simulink model "NDT_Localization"  (R2022a)
settings: Solver=FixedStepAuto  StartTime=0.0  StopTime=10.0  RelTol=1e-3
model workspace (MAT data in the model file):
  SL_ROS_VariableLengthArrays_MaxSizes.CommonInfo.ArrayTruncateAction = 'EmitWarning'
  SL_ROS_VariableLengthArrays_MaxSizes.MsgTypeMap = containers.Map
  SL_ROS_VariableLengthArrays_MaxSizes.MsgTypeMap.serialization.keys = {'sensor_msgs/PointCloud2'}
  SL_ROS_VariableLengthArrays_MaxSizes.MsgTypeMap.serialization.values{1}(1).PropertyName = 'data'
  SL_ROS_VariableLengthArrays_MaxSizes.MsgTypeMap.serialization.values{1}(1).DataType = 'uint8'
  SL_ROS_VariableLengthArrays_MaxSizes.MsgTypeMap.serialization.values{1}(1).MaxLength = 1760000
  SL_ROS_VariableLengthArrays_MaxSizes.MsgTypeMap.serialization.values{1}(2).PropertyName = 'fields'
  SL_ROS_VariableLengthArrays_MaxSizes.MsgTypeMap.serialization.values{1}(2).DataType = 'sensor_msgs/PointField'
  SL_ROS_VariableLengthArrays_MaxSizes.MsgTypeMap.serialization.values{1}(2).MaxLength = 16
  SL_ROS_VariableLengthArrays_MaxSizes.MsgTypeMap.serialization.uniformity = 0
  SL_ROS_VariableLengthArrays_MaxSizes.MsgTypeMap.serialization.keyType = 'char'
  SL_ROS_VariableLengthArrays_MaxSizes.MsgTypeMap.serialization.valueType = 'any'
undefined symbols (not defined in the file or in its folder): null
libraries: ros2lib x9, robotlib x8, simulink x1
(part 1 of 12)
settings Model: Creator=takumi onozawa  LastModifiedBy=takum
settings OptimizationCC: EnhancedBackFolding=on  PassReuseOutputArgsAs=Individual arguments  ZeroExternalMemoryAtStartup=off  ZeroInternalMemoryAtStartup=off  MaxStackSize=64  OptimizeBlockOrder=speed  DifferentSizesBufferReuse=on  OptimizationCustomize=off  EfficientTunableParamExpr=on
settings DebuggingCC: ParameterTunabilityLossMsg=error  UnconnectedInputMsg=warning  UnconnectedOutputMsg=warning  UnconnectedLineMsg=warning
settings SFSimCC: MATLABDynamicMemAlloc=off
settings RTWCC: SystemTargetFile=ert.tlc  HardwareBoard=Robot Operating System 2 (ROS 2)  TLCOptions="-aInlineSetEventsForThisBaseRateFcn=TLC_FALSE -aSuppressMultiTaskScheduler=TLC_FALSE  -aRateBasedStepFcn=0"  TemplateMakefile=ert_default_tmf  Toolchain=Colcon Tools  TargetLang=C++  DLArmComputeVersion=19.05
settings CodeAppCC: ForceParamTrailComments=on  IgnoreCustomStorageClasses=off  OperatorAnnotations=on  SimulinkDataObjDesc=on  SFDataObjDesc=on  InsertBlockDesc=on
settings ERTTargetCC: CodeInterfacePackaging=C++ class  RootIOFormat=Structure reference

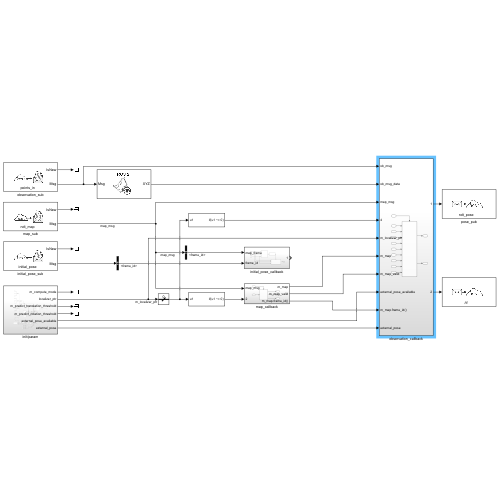
[thumbnail: Simulink's stored preview of the top-level diagram]
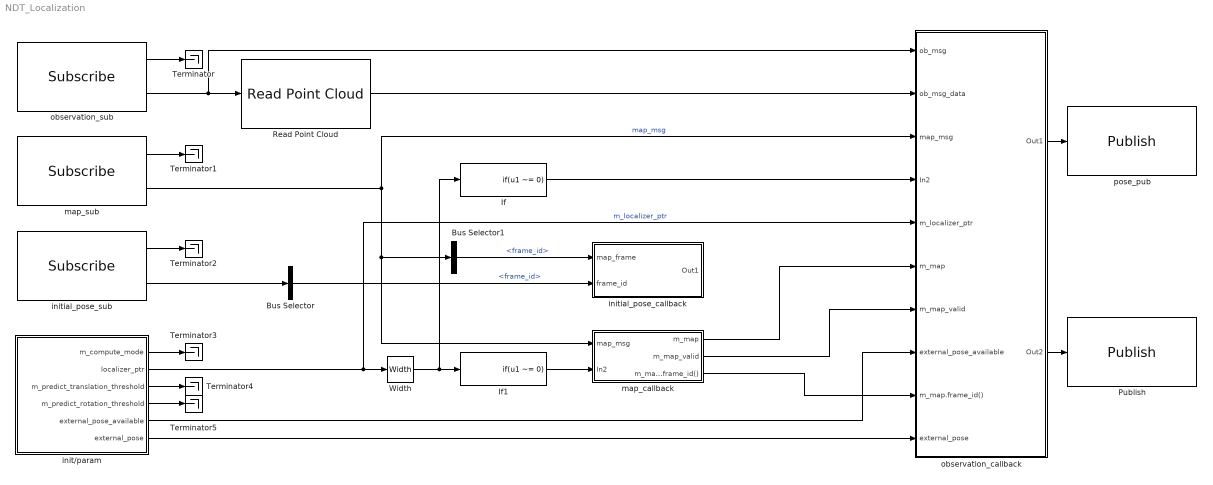
== system NDT_Localization ==
  Bus Selector : BusSelector  OutputSignals=header.frame_id
  Bus Selector1 : BusSelector  OutputSignals=header.frame_id
  If : If  IfExpression=u1 ~= 0  ShowElse=off
  If1 : If  IfExpression=u1 ~= 0  ShowElse=off
  Publish : ros2lib/Publish  topicSource=Specify your own  topic=/tf  messageType=geometry_msgs/Transform  QOSHistory=Keep last  QOSDepth=1  QOSReliability=Reliable  QOSDurability=Volatile
      settings: SourceProductBaseCode=RR
  Read Point Cloud : ros2lib/Read Point Cloud  MaximumPointCloudSize=[480, 640]  PreserveStructure=off  ShowRGBOutput=off  ShowIntensityOutput=off  ShowErrorCodeOutput=off  VariableSizeOutputs=off
      settings: SourceProductBaseCode=RR
  Terminator{,1..5} (6 alike) : Terminator
  Width : Width
  init/param : Subsystem
  initial_pose_callback : Subsystem
  initial_pose_sub : ros2lib/Subscribe  topicSource=Specify your own  topic=initial_pose  messageType=geometry_msgs/PoseWithCovarianceStamped  sampleTime=-1  QOSHistory=Keep last  QOSDepth=1  QOSReliability=Reliable  QOSDurability=Volatile
      settings: SourceProductBaseCode=RR
  map_callback : Subsystem
  map_sub : ros2lib/Subscribe  topicSource=Specify your own  topic=ndt_map  messageType=sensor_msgs/PointCloud2  sampleTime=-1  QOSHistory=Keep last  QOSDepth=1  QOSReliability=Reliable  QOSDurability=Volatile
      settings: SourceProductBaseCode=RR
  observation_callback : Subsystem
  observation_sub : ros2lib/Subscribe  topicSource=Specify your own  topic=points_in  messageType=sensor_msgs/PointCloud2  sampleTime=-1  QOSHistory=Keep last  QOSDepth=1  QOSReliability=Reliable  QOSDurability=Volatile
      settings: SourceProductBaseCode=RR
  pose_pub : ros2lib/Publish  topicSource=Specify your own  topic=ndt_pose  messageType=geometry_msgs/PoseWithCovarianceStamped  QOSHistory=Keep last  QOSDepth=1  QOSReliability=Reliable  QOSDurability=Volatile
      settings: SourceProductBaseCode=RR
  wires:
  observation_sub/1 -> Terminator/1
  map_sub/1 -> Terminator1/1
  initial_pose_sub/1 -> Terminator2/1
  observation_sub/2 -> observation_callback/1(ob_msg), Read Point Cloud/1
  init/param/2(localizer_ptr) -> observation_callback/5(m_localizer_ptr), Width/1  "m_localizer_ptr"
  initial_pose_sub/2 -> Bus Selector/1
  map_sub/2 -> observation_callback/3(map_msg), Bus Selector1/1, map_callback/1(map_msg)  "map_msg"
  Bus Selector1/1 -> initial_pose_callback/1(map_frame)  "<frame_id>"
  Bus Selector/1 -> initial_pose_callback/2(frame_id)  "<frame_id>"
  Read Point Cloud/1 -> observation_callback/2(ob_msg_data)
  If1/1 -> map_callback/2(In2)
  Width/1 -> If/1, If1/1
  If/1 -> observation_callback/4(In2)
  map_callback/2(m_map_valid) -> observation_callback/7(m_map_valid)
  init/param/5(external_pose_available) -> observation_callback/8(external_pose_available)
  init/param/6(external_pose) -> observation_callback/10(external_pose)
  observation_callback/1(Out1) -> pose_pub/1
  map_callback/1(m_map) -> observation_callback/6(m_map)
  observation_callback/2(Out2) -> Publish/1
  map_callback/3(m_map.frame_id()) -> observation_callback/9(m_map.frame_id())
  init/param/1(m_compute_mode) -> Terminator3/1
  init/param/3(m_predict_translation_threshold) -> Terminator4/1
  init/param/4(m_predict_rotation_threshold) -> Terminator5/1

== system NDT_Localization/init//param ==
  Blank Message : ros2lib/Blank Message  messageClass=Message  entityType=geometry_msgs/TransformStamped  messageType=geometry_msgs/TransformStamped  SampleTime=inf
      settings: SourceProductBaseCode=RR
  Bus Creator{,1..2,4..5,8..9} (7 alike) : BusCreator  Inputs=3
  Bus Creator10 : BusCreator  Inputs=4
  Bus Creator11 : BusCreator  Inputs=2
  Bus Creator12 : BusCreator  Inputs=4
  Bus Creator3 : BusCreator  Inputs=4
  Bus Creator6 : BusCreator  Inputs=6
  Bus Creator7 : BusCreator  Inputs=2
  Bus Selector : BusSelector  OutputSignals=header.stamp,header.frame_id_SL_Info,child_frame_id_SL_Info
  Constant{,1..5} (6 alike) : Constant  Value=0
  Constant6 : Constant
  Data Type Conversion : DataTypeConversion  OutDataTypeStr=double  SaturateOnIntegerOverflow=off  RndMeth=Floor
  If : If  NumInputs=5  IfExpression=u2 >= 0 & u1 >= u2 & (u3 >= 0.0 & u3 <= 1.0) & (u4 >= 0.0 & u4 <= 1.0) & u5 >= 1  ShowElse=off
  If Action Subsystem : Subsystem  TreatAsAtomicUnit=on
  MoreThuenteLineSearch : Subsystem
  String Constant : StringConstant  String="\"map\""
  String Constant1 : StringConstant  String="\"base_link\""
  String to ASCII : StringToASCII
  String to ASCII1 : StringToASCII
  guess_time_tolerance_ms : Constant  Value=5  OutDataTypeStr=uint64
  m_external_pose_available : Constant  Value=true  OutDataTypeStr=boolean
  map_capacity : Constant  Value=55000  OutDataTypeStr=uint32
  map_max_point_x : Constant  Value=130.0  OutDataTypeStr=int64
  map_max_point_y : Constant  Value=130.0  OutDataTypeStr=int64
  map_max_point_z : Constant  Value=3.0  OutDataTypeStr=int64
  map_min_point_x : Constant  Value=-130.0  OutDataTypeStr=int64
  map_min_point_y : Constant  Value=-130.0  OutDataTypeStr=int64
  map_min_point_z : Constant  Value=-3.0  OutDataTypeStr=int64
  map_voxel_size_x : Constant  Value=2.0  OutDataTypeStr=int64
  map_voxel_size_y : Constant  Value=2.0  OutDataTypeStr=int64
  map_voxel_size_z : Constant  Value=2.0  OutDataTypeStr=int64
  optimizer_options : Subsystem
  outlier_ratio : Constant  Value=0.55  OutDataTypeStr=double
  predict_rotation_threshold : Constant  Value=0.1
  predict_translation_threshold : Constant  Value=0.5
  scan_capacity : Constant  Value=55000  OutDataTypeStr=uint32
  step_max : Constant  Value=0.12
  step_min : Constant  Value=0.0001
  m_compute_mode : Outport
  localizer_ptr : Outport  Port=2
  m_predict_translation_threshold : Outport  Port=3
  m_predict_rotation_threshold : Outport  Port=4
  external_pose_available : Outport  Port=5
  external_pose : Outport  Port=6
  wires:
  map_voxel_size_x/1 -> Bus Creator2/1  "x"
  Bus Creator/1 -> Bus Creator3/1  "min_point"
  Data Type Conversion/1 -> If/5
  map_min_point_y/1 -> Bus Creator/2  "y"
  Bus Creator1/1 -> Bus Creator3/2  "max_point"
  MoreThuenteLineSearch/1(optimization_direction1) -> Bus Creator6/3
  Bus Creator4/1 -> Bus Creator8/1  "localizer_config"
  map_voxel_size_y/1 -> Bus Creator2/2  "y"
  Bus Creator2/1 -> Bus Creator3/3  "voxel_size"
  map_max_point_x/1 -> Bus Creator1/1  "x"
  step_max/1 -> If/1, Bus Creator6/1  "max_step"
  map_max_point_z/1 -> Bus Creator1/3  "z"
  MoreThuenteLineSearch/2(mu1) -> If/3, Bus Creator6/4
  step_min/1 -> If/2, Bus Creator6/2  "min_step"
  map_min_point_z/1 -> Bus Creator/3  "z"
  map_capacity/1 -> Bus Creator3/4  "capacity"
  MoreThuenteLineSearch/3(eta2) -> Bus Creator6/5, If/4
  optimizer_options/1(optimizer_options) -> Bus Creator7/2  "optimizer_options"
  outlier_ratio/1 -> Bus Creator8/3  "outlier_ratio"
  Bus Creator3/1 -> Bus Creator4/1  "map_config"
  predict_rotation_threshold/1 -> m_predict_rotation_threshold/1  "predict_rotation_threshold"
  map_max_point_y/1 -> Bus Creator1/2  "y"
  guess_time_tolerance_ms/1 -> Bus Creator4/3  "milliseconds"
  map_voxel_size_z/1 -> Bus Creator2/3  "z"
  predict_translation_threshold/1 -> m_predict_translation_threshold/1  "predict_translation_threshold"
  MoreThuenteLineSearch/4(max_iterations1) -> Bus Creator6/6, Data Type Conversion/1
  If/1 -> If Action Subsystem/Action
  Bus Creator6/1 -> Bus Creator7/1  "MoreThuenteLineSearch"
  Bus Creator7/1 -> Bus Creator8/2  "OptimizerT"
  scan_capacity/1 -> Bus Creator4/2  "capacity"
  map_min_point_x/1 -> Bus Creator/1  "x"
  Bus Creator8/1 -> localizer_ptr/1  "localizer_ptr"
  If Action Subsystem/1(m_compute_mode) -> m_compute_mode/1  "m_compute_mode"
  m_external_pose_available/1 -> external_pose_available/1
  Blank Message/1 -> Bus Selector/1
  Bus Selector/1 -> Bus Creator5/1  "<stamp>"
  String to ASCII/1 -> Bus Creator5/2  "frame_id"
  Bus Selector/2 -> Bus Creator5/3  "<frame_id_SL_Info>"
  Bus Creator5/1 -> Bus Creator12/1  "header"
  String to ASCII1/1 -> Bus Creator12/2  "child_frame_id"
  Bus Selector/3 -> Bus Creator12/3  "<child_frame_id_SL_Info>"
  Constant/1 -> Bus Creator9/1  "x"
  Constant1/1 -> Bus Creator9/2  "y"
  Constant2/1 -> Bus Creator9/3  "z"
  Bus Creator9/1 -> Bus Creator11/1  "translation"
  Constant3/1 -> Bus Creator10/1  "x"
  Constant4/1 -> Bus Creator10/2  "y"
  Constant5/1 -> Bus Creator10/3  "z"
  Constant6/1 -> Bus Creator10/4  "w"
  Bus Creator10/1 -> Bus Creator11/2  "rotation"
  Bus Creator11/1 -> Bus Creator12/4  "transform"
  String Constant1/1 -> String to ASCII1/1
  String Constant/1 -> String to ASCII/1
  Bus Creator12/1 -> external_pose/1  "external_pose"

== system NDT_Localization/initial_pose_callback ==
  map_frame : Inport
  frame_id : Inport  Port=2
  If1 : If  IfExpression=u1 ~= 0  ShowElse=off
  TimePointZero : Constant  Value=0
  canTransform : Subsystem
  lookupTransform : Subsystem  TreatAsAtomicUnit=on
  Out1 : Outport
  wires:
  lookupTransform/1(Out1) -> Out1/1
  canTransform/1(<frame_id>) -> If1/1
  If1/1 -> lookupTransform/Action
  map_frame/1 -> lookupTransform/1(target_frame), canTransform/1(target_frame)
  TimePointZero/1 -> lookupTransform/3(time), canTransform/3(time)
  frame_id/1 -> lookupTransform/2(source_frame), canTransform/2(source_frame)

== system NDT_Localization/map_callback ==
  map_msg : Inport
  In2 : Inport  Port=2
  check_localizer : Subsystem  TreatAsAtomicUnit=on
  m_map : Outport
  m_map_valid : Outport  Port=2
  m_map.frame_id() : Outport  Port=3
  wires:
  map_msg/1 -> check_localizer/1(map_msg)
  In2/1 -> check_localizer/Action
  check_localizer/1(m_map) -> m_map/1
  check_localizer/2(m_map_valid) -> m_map_valid/1
  check_localizer/3(m_map.frame_id()) -> m_map.frame_id()/1

== system NDT_Localization/observation_callback ==
  ob_msg : Inport
  ob_msg_data : Inport  Port=2
  map_msg : Inport  Port=3
  In2 : Inport  Port=4
  m_localizer_ptr : Inport  Port=5
  m_map : Inport  Port=6
  m_map_valid : Inport  Port=7
  external_pose_available : Inport  Port=8
  m_map.frame_id() : Inport  Port=9
  external_pose : Inport  Port=10
  check_localizer : Subsystem  TreatAsAtomicUnit=on
  Out1 : Outport
  Out2 : Outport  Port=2
  wires:
  In2/1 -> check_localizer/Action
  check_localizer/1(Out1) -> Out1/1
  m_map_valid/1 -> check_localizer/1(m_map_valid)
  ob_msg/1 -> check_localizer/2(ob_msg)
  map_msg/1 -> check_localizer/4(map_msg)
  external_pose_available/1 -> check_localizer/5(external_pose_available)
  external_pose/1 -> check_localizer/6(external_pose)
  m_map/1 -> check_localizer/7(m_map)
  check_localizer/2(Out2) -> Out2/1
  m_localizer_ptr/1 -> check_localizer/9(m_localizer_ptr)
  m_map.frame_id()/1 -> check_localizer/8(m_map.frame_id())
  ob_msg_data/1 -> check_localizer/3(ob_msg_data)

== system NDT_Localization/init//param/If Action Subsystem ==
  Action Port : ActionPort  ActionPortLabel=if(u2 >= 0 & u1 >= u2 & (u3 >= 0.0 & u3 <= 1.0) & (u4 >= 0.0 & u4 <= 1.0) & u5 >= 1)
  Bus Creator : BusCreator  Inputs=2
  set_jacobian : MATLAB Function  TreatAsAtomicUnit=on
  set_score : Constant  Value=0.0  OutDataTypeStr=single
  m_compute_mode : Outport
  wires:
  Bus Creator/1 -> m_compute_mode/1
  set_score/1 -> Bus Creator/1
  set_jacobian/1(jacobian) -> Bus Creator/2

== system NDT_Localization/init//param/MoreThuenteLineSearch ==
  eta : Constant  Value=0.1  OutDataTypeStr=double
  max_iterations : Constant  Value=10  OutDataTypeStr=int32
  mu : Constant  Value=0.0001
  optimization_direction : Constant  Value=1.0  OutDataTypeStr=double
  optimization_direction1 : Outport
  mu1 : Outport  Port=2
  eta2 : Outport  Port=3
  max_iterations1 : Outport  Port=4
  wires:
  optimization_direction/1 -> optimization_direction1/1  "optimization_direction"
  max_iterations/1 -> max_iterations1/1  "max_iterations"
  mu/1 -> mu1/1  "mu"
  eta/1 -> eta2/1  "eta"

== system NDT_Localization/init//param/optimizer_options ==
  Bus Creator5 : BusCreator  Inputs=4
  gradient_tolerance : Constant  Value=0.001  OutDataTypeStr=double
  max_iterations : Constant  Value=50  OutDataTypeStr=uint64
  parameter_tolerance : Constant  Value=0.001  OutDataTypeStr=double
  score_tolerance : Constant  Value=0.001  OutDataTypeStr=double
  optimizer_options : Outport
  wires:
  gradient_tolerance/1 -> Bus Creator5/4  "gradient_tolerance"
  parameter_tolerance/1 -> Bus Creator5/3  "parameter_tolerance"
  score_tolerance/1 -> Bus Creator5/2  "score_tolerance"
  Bus Creator5/1 -> optimizer_options/1  "optimizer_options"
  max_iterations/1 -> Bus Creator5/1  "max_iterations"

== system NDT_Localization/initial_pose_callback/canTransform ==
  target_frame : Inport
  source_frame : Inport  Port=2
  time : Inport  Port=3
  Bus Selector : BusSelector  OutputSignals=header.frame_id
  Constant : Constant  Value=true  OutDataTypeStr=boolean
  Constant1 : Constant  Value=false  OutDataTypeStr=boolean
  Constant2 : Constant  Value=false  OutDataTypeStr=boolean
  Constant3 : Constant  Value=false  OutDataTypeStr=boolean
  If1 : If  NumInputs=4  IfExpression=u1 == 1  ElseIfExpressions=u2 ~= 0, u3 == 0, u4 == 0
  Merge : Merge  Inputs=5
  String Compare : StringCompare
  else : Subsystem  TreatAsAtomicUnit=on
  lookupFrameNumber : Subsystem
  lookupFrameNumber1 : Subsystem
  true : Subsystem  TreatAsAtomicUnit=on
  true1 : Subsystem  TreatAsAtomicUnit=on
  true2 : Subsystem  TreatAsAtomicUnit=on
  true3 : Subsystem  TreatAsAtomicUnit=on
  warnFrameId : Subsystem
  <frame_id> : Outport
  wires:
  true/1(Out1) -> Merge/1
  true2/1(Out1) -> Merge/3
  Merge/1 -> <frame_id>/1
  else/1(Out1) -> Merge/5
  If1/5 -> else/Action
  Constant2/1 -> true2/1(In1)
  If1/3 -> true2/Action
  If1/4 -> true3/Action
  true1/1(Out1) -> Merge/2
  If1/2 -> true1/Action
  lookupFrameNumber1/1(source_id) -> else/2(source_id), If1/4  "source_id"
  Constant3/1 -> true3/1(In1)
  warnFrameId/1(Out1) -> If1/2
  String Compare/1 -> If1/1
  lookupFrameNumber/1(target_id) -> else/1(target_id), If1/3  "target_id"
  Constant1/1 -> true1/1(In1)
  Constant/1 -> true/1(In1)
  true3/1(Out1) -> Merge/4
  If1/1 -> true/Action
  target_frame/1 -> Bus Selector/1
  source_frame/1 -> lookupFrameNumber1/1(source_frame), warnFrameId/2(frame_id), String Compare/2
  time/1 -> else/3(time)
  Bus Selector/1 -> String Compare/1, warnFrameId/1(map_frame), lookupFrameNumber/1(target_frame)  "<frame_id>"

== system NDT_Localization/initial_pose_callback/lookupTransform ==
  target_frame : Inport
  source_frame : Inport  Port=2
  time : Inport  Port=3
  Action Port : ActionPort  ActionPortLabel=if(u1 ~= 0)
  If : If  IfExpression=u1 ~= 0
  String Compare : StringCompare
  Switch : Switch  Criteria=u2 > Threshold  SaturateOnIntegerOverflow=off  InputSameDT=off
  if_false : Subsystem  TreatAsAtomicUnit=on
  if_true : Subsystem  TreatAsAtomicUnit=on
  Out1 : Outport
  wires:
  source_frame/1 -> String Compare/2, if_false/2(source_frame), if_true/2(source_frame)
  String Compare/1 -> Switch/2, If/1
  If/1 -> if_true/Action
  If/2 -> if_false/Action
  time/1 -> if_false/3(time), if_true/3(time)
  target_frame/1 -> String Compare/1, if_false/1(target_frame), if_true/1(target_frame)
  if_true/1(identity) -> Switch/1
  if_false/1(output_transform) -> Switch/3
  Switch/1 -> Out1/1

== system NDT_Localization/map_callback/check_localizer ==
  map_msg : Inport
  Action Port : ActionPort  ActionPortLabel=if(u1 ~= 0)
  set_map : Subsystem
  m_map : Outport
  m_map_valid : Outport  Port=2
  m_map.frame_id() : Outport  Port=3
  wires:
  map_msg/1 -> set_map/1(msg)
  set_map/1(impl()) -> m_map/1
  set_map/2(m_map_valid) -> m_map_valid/1
  set_map/3(m_map.frame_id()) -> m_map.frame_id()/1

== system NDT_Localization/observation_callback/check_localizer ==
  m_map_valid : Inport
  ob_msg : Inport  Port=2
  ob_msg_data : Inport  Port=3
  map_msg : Inport  Port=4
  external_pose_available : Inport  Port=5
  external_pose : Inport  Port=6
  m_map : Inport  Port=7
  m_map.frame_id() : Inport  Port=8
  m_localizer_ptr : Inport  Port=9
  Action Port : ActionPort  ActionPortLabel=if(u1 ~= 0)
  Data Type Conversion : DataTypeConversion  OutDataTypeStr=uint8  SaturateOnIntegerOverflow=off  RndMeth=Floor
  If : If  IfExpression=u1 ~= 0  ShowElse=off
  If Action Subsystem : Subsystem  TreatAsAtomicUnit=on
  If Action Subsystem1 : Subsystem  TreatAsAtomicUnit=on
  If Action Subsystem2 : Subsystem  TreatAsAtomicUnit=on
  If1 : If  IfExpression=u1 ~= 0
  Merge : Merge
  Out1 : Outport
  Out2 : Outport  Port=2
  wires:
  m_map_valid/1 -> Data Type Conversion/1
  Data Type Conversion/1 -> If/1
  If/1 -> If Action Subsystem/Action
  ob_msg/1 -> If Action Subsystem/1(ob_msg)
  map_msg/1 -> If Action Subsystem/3(map_msg)
  external_pose_available/1 -> If Action Subsystem/4(external_pose_available)
  external_pose/1 -> If Action Subsystem/5(external_pose)
  m_map/1 -> If Action Subsystem/6(m_map)
  If Action Subsystem/3(Out2) -> If1/1
  If Action Subsystem1/1(Out1) -> Out1/1
  If1/1 -> If Action Subsystem1/Action
  If1/2 -> If Action Subsystem2/Action
  If Action Subsystem/2(pose_out) -> If Action Subsystem1/2(pose_out), Merge/1
  If Action Subsystem2/1(Out1) -> Merge/2
  If Action Subsystem/4(msg.header.stamp) -> If Action Subsystem2/1(msg.header.stamp)
  m_localizer_ptr/1 -> If Action Subsystem2/2(m_localizer_ptr), If Action Subsystem/8(localizer_ptr)
  Merge/1 -> Out2/1
  If Action Subsystem/1(msg) -> If Action Subsystem1/1(msg)
  m_map.frame_id()/1 -> If Action Subsystem/7(m_map.frame_id())
  ob_msg_data/1 -> If Action Subsystem/2(ob_msg_data)

== system NDT_Localization/initial_pose_callback/canTransform/else ==
  target_id : Inport
  source_id : Inport  Port=2
  time : Inport  Port=3
  Action Port : ActionPort  ActionPortLabel=else
  canTransformNoLock : Subsystem
  Out1 : Outport
  wires:
  source_id/1 -> canTransformNoLock/2(source_id)
  target_id/1 -> canTransformNoLock/1(target_id)
  canTransformNoLock/1(Out1) -> Out1/1
  time/1 -> canTransformNoLock/3(time)

== system NDT_Localization/initial_pose_callback/canTransform/lookupFrameNumber ==
  target_frame : Inport
  Cast : DataTypeConversion  SaturateOnIntegerOverflow=off  RndMeth=Floor
  target_id : Outport
  wires:
  target_frame/1 -> Cast/1
  Cast/1 -> target_id/1

== system NDT_Localization/initial_pose_callback/canTransform/lookupFrameNumber1 ==
  source_frame : Inport
  Cast : DataTypeConversion  SaturateOnIntegerOverflow=off  RndMeth=Floor
  source_id : Outport
  wires:
  Cast/1 -> source_id/1
  source_frame/1 -> Cast/1

== system NDT_Localization/initial_pose_callback/canTransform/true ==
  In1 : Inport
  Action Port : ActionPort  ActionPortLabel=if(u1 == 1)
  Out1 : Outport
  wires:
  In1/1 -> Out1/1

== system NDT_Localization/initial_pose_callback/canTransform/true1 ==
  In1 : Inport
  Action Port : ActionPort  ActionPortLabel=elseif(u2 ~= 0)
  Out1 : Outport
  wires:
  In1/1 -> Out1/1

== system NDT_Localization/initial_pose_callback/canTransform/true2 ==
  In1 : Inport
  Action Port : ActionPort  ActionPortLabel=elseif( u3 == 0)
  Out1 : Outport
  wires:
  In1/1 -> Out1/1

== system NDT_Localization/initial_pose_callback/canTransform/true3 ==
  In1 : Inport
  Action Port : ActionPort  ActionPortLabel=elseif( u4 == 0)
  Out1 : Outport
  wires:
  In1/1 -> Out1/1

== system NDT_Localization/initial_pose_callback/canTransform/warnFrameId ==
  map_frame : Inport
  frame_id : Inport  Port=2
  Add : Sum
  Add1 : Sum  Inputs=+++
  Cast : DataTypeConversion  OutDataTypeStr=boolean  SaturateOnIntegerOverflow=off  RndMeth=Floor
  Constant : Constant  OutDataTypeStr=double
  Display : Display
  If1 : If  IfExpression=u1 == 0  ShowElse=off
  If2 : If  IfExpression=u1 == 0  ShowElse=off
  If3 : If  ShowElse=off
  String Compare : StringCompare  CompareOption=First N characters
  String Compare1 : StringCompare  CompareOption=First N characters
  String Constant : StringConstant  String="\"\\\""
  String Length : StringLength
  String Length1 : StringLength
  false1 : Subsystem  TreatAsAtomicUnit=on
  false2 : Subsystem  TreatAsAtomicUnit=on
  false3 : Subsystem  TreatAsAtomicUnit=on
  Out1 : Outport
  wires:
  false2/1(Out1) -> Add1/2
  Constant/1 -> false1/1(In1), false3/1(In1), false2/1(In1)
  If1/1 -> false1/Action
  false3/1(Out1) -> Add1/3
  Add1/1 -> Cast/1
  String Constant/1 -> String Compare/2, String Compare1/1
  String Compare/1 -> Add/1
  String Compare1/1 -> Add/2
  Add/1 -> If3/1
  map_frame/1 -> String Compare/1, String Length/1
  false1/1(Out1) -> Add1/1
  frame_id/1 -> String Compare1/2, String Length1/1
  String Length/1 -> If1/1
  If3/1 -> false2/Action
  If2/1 -> false3/Action
  String Length1/1 -> If2/1
  Cast/1 -> Out1/1, Display/1

== system NDT_Localization/initial_pose_callback/lookupTransform/if_false ==
  target_frame : Inport
  source_frame : Inport  Port=2
  time : Inport  Port=3
  Action Port : ActionPort  ActionPortLabel=else
  Bus Creator : BusCreator  Inputs=3
  Bus Creator1 : BusCreator  Inputs=3
  Bus Creator2 : BusCreator  Inputs=2
  Bus Creator3 : BusCreator  Inputs=3
  Bus Creator4 : BusCreator  Inputs=4
  Bus Selector : BusSelector  OutputSignals=time,result_vec.x,result_vec.y,result_vec.z,result_quat.x,result_quat.y,result_quat.z,result_quat.w
  Constant : Constant
  Subsystem : Subsystem
  lookupFrameNumber : Subsystem
  lookupFrameNumber1 : Subsystem
  walkToTopParent : Subsystem  Commented=on
  output_transform : Outport
  wires:
  target_frame/1 -> lookupFrameNumber/1(target_frame), Bus Creator1/3  "frame_id"
  lookupFrameNumber/1(target_id) -> walkToTopParent/3(target_id)
  lookupFrameNumber1/1(source_id) -> walkToTopParent/4(source_id)
  time/1 -> walkToTopParent/2(time)
  Subsystem/1(accum) -> Bus Selector/1, walkToTopParent/1(accum)
  Constant/1 -> Bus Creator1/1  "sec"
  source_frame/1 -> Bus Creator/2, lookupFrameNumber1/1(source_frame)  "child_frame_id"
  Bus Selector/6 -> Bus Creator4/2  "<y>"
  Bus Creator3/1 -> Bus Creator2/1  "translation"
  Bus Selector/8 -> Bus Creator4/4  "<w>"
  Bus Creator4/1 -> Bus Creator2/2  "rotation"
  Bus Creator2/1 -> Bus Creator/3  "transform"
  Bus Creator1/1 -> Bus Creator/1  "header"
  Bus Selector/3 -> Bus Creator3/2  "<y>"
  Bus Selector/5 -> Bus Creator4/1  "<x>"
  Bus Selector/7 -> Bus Creator4/3  "<z>"
  Bus Creator/1 -> output_transform/1
  Bus Selector/1 -> Bus Creator1/2  "<time>"
  Bus Selector/2 -> Bus Creator3/1  "<x>"
  Bus Selector/4 -> Bus Creator3/3  "<z>"

== system NDT_Localization/initial_pose_callback/lookupTransform/if_true ==
  target_frame : Inport
  source_frame : Inport  Port=2
  time : Inport  Port=3
  Action Port : ActionPort  ActionPortLabel=if(u1 ~= 0)
  Bus Creator : BusCreator  Inputs=3
  Bus Creator1 : BusCreator  Inputs=3
  Bus Creator2 : BusCreator  Inputs=2
  Bus Creator3 : BusCreator  Inputs=3
  Bus Creator4 : BusCreator  Inputs=4
  Constant : Constant  Value=false  OutDataTypeStr=boolean
  If : If  NumInputs=2  IfExpression=u1 == u2
  If Action Subsystem : Subsystem  TreatAsAtomicUnit=on
  If Action Subsystem1 : Subsystem  TreatAsAtomicUnit=on
  MATLAB Function : MATLAB Function  TreatAsAtomicUnit=on
  Merge : Merge
  Switch : Switch  Criteria=u2 > Threshold  SaturateOnIntegerOverflow=off  InputSameDT=off
  getFrame : Subsystem
  getLatestTimestamp : Subsystem
  lookupFrameNumber : Subsystem
  sec : Constant  Value=0  OutDataTypeStr=uint32
  w : Constant  OutDataTypeStr=single
  x : Constant  Value=0  OutDataTypeStr=single
  x1 : Constant  Value=0  OutDataTypeStr=single
  y : Constant  Value=0  OutDataTypeStr=single
  y1 : Constant  Value=0  OutDataTypeStr=single
  z : Constant  Value=0  OutDataTypeStr=single
  z1 : Constant  Value=0  OutDataTypeStr=single
  identity : Outport
  wires:
  Bus Creator1/1 -> Bus Creator/1  "header"
  sec/1 -> Bus Creator1/1  "sec"
  Bus Creator/1 -> identity/1
  source_frame/1 -> Bus Creator/2  "child_frame_id"
  Bus Creator2/1 -> Bus Creator/3  "transform"
  Bus Creator3/1 -> Bus Creator2/1  "translation"
  Bus Creator4/1 -> Bus Creator2/2  "rotation"
  Switch/1 -> Bus Creator1/2  "stamp"
  target_frame/1 -> Bus Creator1/3, lookupFrameNumber/1(target_frame)  "frame_id"
  x/1 -> Bus Creator3/1  "x"
  y/1 -> Bus Creator3/2  "y"
  z/1 -> Bus Creator3/3  "z"
  z1/1 -> Bus Creator4/3  "z"
  y1/1 -> Bus Creator4/2  "y"
  x1/1 -> Bus Creator4/1  "x"
  w/1 -> Bus Creator4/4  "w"
  time/1 -> Switch/3, If/1
  MATLAB Function/1(now) -> If/2
  If/2 -> If Action Subsystem/Action
  If/1 -> If Action Subsystem1/Action
  If Action Subsystem1/1(out1) -> Merge/1
  If Action Subsystem/1(Out1) -> Merge/2
  Merge/1 -> Switch/2
  Constant/1 -> If Action Subsystem/1(In1)
  lookupFrameNumber/1(target_id) -> getFrame/1(target_id)
  getFrame/1(cache) -> If Action Subsystem1/1(cache), getLatestTimestamp/1(cache)
  getLatestTimestamp/1(LatestTimestamp) -> Switch/1

== system NDT_Localization/map_callback/check_localizer/set_map ==
  msg : Inport
  Switch : Switch  Criteria=u2 ~= 0  SaturateOnIntegerOverflow=off  InputSameDT=off
  Terminator : Terminator
  set_map_impl : Subsystem
  set_map_invalid() : Constant  Value=false
  set_map_valid() : Constant  Value=true
  impl() : Outport
  m_map_valid : Outport  Port=2
  m_map.frame_id() : Outport  Port=3
  wires:
  msg/1 -> set_map_impl/1(msg)
  set_map_valid()/1 -> Switch/1
  set_map_invalid()/1 -> Switch/3
  Switch/1 -> m_map_valid/1  "m_map_valid"
  set_map_impl/4(Out1) -> Switch/2
  set_map_impl/1(m_stamp) -> Terminator/1
  set_map_impl/2(m_frame_id) -> m_map.frame_id()/1
  set_map_impl/3(impl()) -> impl()/1

== system NDT_Localization/observation_callback/check_localizer/If Action Subsystem ==
  ob_msg : Inport
  ob_msg_data : Inport  Port=2
  map_msg : Inport  Port=3
  external_pose_available : Inport  Port=4
  external_pose : Inport  Port=5
  m_map : Inport  Port=6
  m_map.frame_id() : Inport  Port=7
  localizer_ptr : Inport  Port=8
  Action Port : ActionPort  ActionPortLabel=if(u1 ~= 0)
  Add : Sum
  Bus Creator : BusCreator  Inputs=4
  Bus Creator1 : BusCreator  Inputs=3
  Bus Selector : BusSelector  OutputSignals=header.stamp,header.stamp.sec,header.stamp.nanosec,header.frame_id
  Bus Selector1 : BusSelector  OutputSignals=header.frame_id
  Bus Selector2 : BusSelector  OutputSignals=header.frame_id,header.frame_id_SL_Info,child_frame_id,child_frame_id_SL_Info,transform
  Constant : Constant  Value=9
  Data Type Conversion : DataTypeConversion  OutDataTypeStr=uint8  SaturateOnIntegerOverflow=off  RndMeth=Floor
  Data Type Conversion1 : DataTypeConversion  OutDataTypeStr=uint8  SaturateOnIntegerOverflow=off  RndMeth=Floor
  If : If  IfExpression=u1 ~= 0
  If Action Subsystem : Subsystem  TreatAsAtomicUnit=on
  If Action Subsystem1 : Subsystem  TreatAsAtomicUnit=on
  If Action Subsystem2 : Subsystem  TreatAsAtomicUnit=on
  If1 : If  IfExpression=u1 ~= 0  ShowElse=off
  Logical Operator1 : Logic  AllPortsSameDT=off  OutDataTypeStr=boolean
  Math Function : Math  Operator=10^u
  Merge : Merge
  Merge2 : Merge  Inputs=3
  Product : Product
  Relational Operator : RelationalOperator  Operator===  OutDataTypeStr=boolean  RndMeth=Simplest  InputSameDT=off
  Relational Operator1 : RelationalOperator  Operator===  OutDataTypeStr=boolean  RndMeth=Simplest  InputSameDT=off
  guess : Subsystem
  register_measurement_impl : Subsystem
  validate_output : Subsystem
  msg : Outport
  pose_out : Outport  Port=2
  Out2 : Outport  Port=3
  msg.header.stamp : Outport  Port=4
  wires:
  ob_msg/1 -> Bus Selector/1, If Action Subsystem/2(ob_msg), register_measurement_impl/2(ob_msg)
  Bus Selector/2 -> Product/1  "<sec>"
  Bus Selector/3 -> Add/2  "<nanosec>"
  Constant/1 -> Math Function/1
  Math Function/1 -> Product/2
  Product/1 -> Add/1
  Add/1 -> guess/1(observation_time), register_measurement_impl/1(observation_time)  "observation_time"
  Bus Selector/4 -> guess/3(observation_frame), Relational Operator1/2  "<frame_id>"
  map_msg/1 -> Bus Selector1/1
  Bus Selector1/1 -> Relational Operator/2, guess/2(map_frame)  "<frame_id>"
  If Action Subsystem/2(Out1) -> pose_out/1
  guess/1(initial_guess) -> If Action Subsystem2/3(initial_guess)  "initial_guess"
  external_pose_available/1 -> If Action Subsystem2/2(external_pose_available)
  Relational Operator/1 -> Logical Operator1/1
  Relational Operator1/1 -> Logical Operator1/2
  Bus Selector2/1 -> Relational Operator/1, Bus Creator1/2  "<frame_id>"
  Bus Selector/1 -> msg.header.stamp/1, Bus Creator1/1  "<stamp>"
  Bus Creator/1 -> If Action Subsystem2/1(In1)  "initial_guess"
  external_pose/1 -> Bus Selector2/1
  Bus Selector2/3 -> Bus Creator/2, Relational Operator1/1  "<child_frame_id>"
  Bus Selector2/2 -> Bus Creator1/3  "<frame_id_SL_Info>"
  Bus Creator1/1 -> Bus Creator/1  "header"
  Bus Selector2/4 -> Bus Creator/3  "<child_frame_id_SL_Info>"
  Bus Selector2/5 -> Bus Creator/4  "<transform>"
  If Action Subsystem2/1(Out1) -> validate_output/3(initial_guess), register_measurement_impl/4(initial_guess)  "initial_guess"
  If/1 -> If Action Subsystem/Action
  register_measurement_impl/1(summary) -> If Action Subsystem/3(summary), validate_output/1(summary)
  register_measurement_impl/2(pose_out) -> If Action Subsystem/1(pose_out), validate_output/2(pose_out)
  Data Type Conversion/1 -> If/1
  validate_output/1(ret_out) -> Data Type Conversion/1
  If/2 -> If Action Subsystem1/Action
  If Action Subsystem/3(Out2) -> Merge/1
  If Action Subsystem1/1(Out1) -> Merge/2
  Merge/1 -> Merge2/3
  Data Type Conversion1/1 -> If1/1
  Logical Operator1/1 -> Data Type Conversion1/1
  If1/1 -> If Action Subsystem2/Action
  If Action Subsystem2/2(Out2) -> Merge2/1
  Merge2/1 -> Out2/1
  register_measurement_impl/3(Out1) -> Merge2/2
  m_map/1 -> register_measurement_impl/5(m_map)
  If Action Subsystem/1(msg) -> msg/1
  m_map.frame_id()/1 -> register_measurement_impl/6(m_map.frame_id())
  ob_msg_data/1 -> register_measurement_impl/3(ob_msg_data)
  localizer_ptr/1 -> register_measurement_impl/7(localizer_ptr)

== system NDT_Localization/observation_callback/check_localizer/If Action Subsystem1 ==
  msg : Inport
  pose_out : Inport  Port=2
  Action Port : ActionPort  ActionPortLabel=if(u1 ~= 0)
  Terminator : Terminator
  Out1 : Outport
  wires:
  pose_out/1 -> Out1/1
  msg/1 -> Terminator/1

== system NDT_Localization/observation_callback/check_localizer/If Action Subsystem2 ==
  msg.header.stamp : Inport
  m_localizer_ptr : Inport  Port=2
  Action Port : ActionPort  ActionPortLabel=else
  republish_tf : Subsystem
  Out1 : Outport
  wires:
  republish_tf/1(Out1) -> Out1/1
  m_localizer_ptr/1 -> republish_tf/2(m_localizer_ptr)
  msg.header.stamp/1 -> republish_tf/1(msg.header.stamp)

== system NDT_Localization/initial_pose_callback/canTransform/else/canTransformNoLock ==
  target_id : Inport
  source_id : Inport  Port=2
  time : Inport  Port=3
  Constant : Constant  Value=true  OutDataTypeStr=boolean
  If : If  NumInputs=2  IfExpression=u1 == u2
  Merge : Merge
  true : Subsystem  TreatAsAtomicUnit=on
  walkToTopParent : Subsystem  TreatAsAtomicUnit=on
  Out1 : Outport
  wires:
  source_id/1 -> walkToTopParent/4(source_id), If/2  "source_id"
  target_id/1 -> walkToTopParent/3(target_id), If/1  "target_id"
  If/1 -> true/Action
  Constant/1 -> true/1(In1)
  If/2 -> walkToTopParent/Action
  walkToTopParent/1(Out2) -> Merge/2
  true/1(Out1) -> Merge/1
  Merge/1 -> Out1/1
  time/1 -> walkToTopParent/2(time)

== system NDT_Localization/initial_pose_callback/canTransform/warnFrameId/false1 ==
  In1 : Inport
  Action Port : ActionPort  ActionPortLabel=if(u1 == 0)
  Out1 : Outport
  wires:
  In1/1 -> Out1/1

== system NDT_Localization/initial_pose_callback/canTransform/warnFrameId/false2 ==
  In1 : Inport
  Action Port : ActionPort  ActionPortLabel=if(u1 > 0)
  Out1 : Outport
  wires:
  In1/1 -> Out1/1

== system NDT_Localization/initial_pose_callback/canTransform/warnFrameId/false3 ==
  In1 : Inport
  Action Port : ActionPort  ActionPortLabel=if(u1 == 0)
  Out1 : Outport
  wires:
  In1/1 -> Out1/1

== system NDT_Localization/initial_pose_callback/lookupTransform/if_false/Subsystem ==
  Bus Creator : BusCreator  Inputs=8
  Bus Creator1 : BusCreator  Inputs=5
  Bus Creator{2,4,6,9} (4 alike) : BusCreator  Inputs=4  OutDataTypeStr=Bus: SL_Bus_geometry_msgs_Quaternion
      settings: InheritFromInputs=off
  Bus Creator{3,5,7..8} (4 alike) : BusCreator  Inputs=3  OutDataTypeStr=Bus: SL_Bus_geometry_msgs_Vector3
      settings: InheritFromInputs=off
  Constant : Constant  OutDataTypeStr=uint32
  Constant1 : Constant  OutDataTypeStr=uint32
  Current Time : robotlib/Current Time  Commented=on  OutputFormat=bus  SampleTime=-1  ModelName=robotlib
      settings: SourceProductBaseCode=RR
  Current Time1 : robotlib/Current Time  Commented=on  OutputFormat=bus  SampleTime=-1  ModelName=robotlib
      settings: SourceProductBaseCode=RR
  w{,1..3} (4 alike) : Constant  OutDataTypeStr=single
  x{,1..7} (8 alike) : Constant  Value=0  OutDataTypeStr=single
  y{,1..7} (8 alike) : Constant  Value=0  OutDataTypeStr=single
  z{,1..7} (8 alike) : Constant  Value=0  OutDataTypeStr=single
  accum : Outport
  wires:
  Bus Creator3/1 -> Bus Creator/4  "source_to_top_vec"
  z4/1 -> Bus Creator6/3  "z"
  z7/1 -> Bus Creator9/3  "z"
  y7/1 -> Bus Creator9/2  "y"
  z1/1 -> Bus Creator4/3  "z"
  y6/1 -> Bus Creator8/2  "y"
  z3/1 -> Bus Creator5/3  "z"
  y1/1 -> Bus Creator4/2  "y"
  w3/1 -> Bus Creator9/4  "w"
  Constant1/1 -> Bus Creator1/5  "child_frame_id_"
  z6/1 -> Bus Creator8/3  "z"
  w/1 -> Bus Creator4/4  "w"
  y/1 -> Bus Creator3/2  "y"
  Bus Creator5/1 -> Bus Creator/6  "terget_to_top_vec"
  y3/1 -> Bus Creator5/2  "y"
  x6/1 -> Bus Creator8/1  "x"
  y4/1 -> Bus Creator6/2  "y"
  Bus Creator6/1 -> Bus Creator/7  "result_quat"
  Bus Creator1/1 -> Bus Creator/1  "st"
  Current Time/1 -> Bus Creator/2  "time"
  x7/1 -> Bus Creator9/1  "x"
  Bus Creator8/1 -> Bus Creator1/2  "translation_"
  Constant/1 -> Bus Creator1/4  "frame_id_"
  y2/1 -> Bus Creator2/2  "y"
  w2/1 -> Bus Creator6/4  "w"
  z2/1 -> Bus Creator2/3  "z"
  Bus Creator4/1 -> Bus Creator/3  "source_to_top_quat"
  x1/1 -> Bus Creator4/1  "x"
  x4/1 -> Bus Creator6/1  "x"
  z/1 -> Bus Creator3/3  "z"
  y5/1 -> Bus Creator7/2  "y"
  x2/1 -> Bus Creator2/1  "x"
  x5/1 -> Bus Creator7/1  "x"
  z5/1 -> Bus Creator7/3  "z"
  Bus Creator7/1 -> Bus Creator/8  "result_vec"
  w1/1 -> Bus Creator2/4  "w"
  x/1 -> Bus Creator3/1  "x"
  Bus Creator2/1 -> Bus Creator/5  "target_to_top_quat"
  Bus Creator9/1 -> Bus Creator1/1  "rotation_"
  Bus Creator/1 -> accum/1  "accum"
  x3/1 -> Bus Creator5/1  "x"
  Current Time1/1 -> Bus Creator1/3  "stamp_"

== system NDT_Localization/initial_pose_callback/lookupTransform/if_false/lookupFrameNumber ==
  target_frame : Inport
  Cast : DataTypeConversion  OutDataTypeStr=uint32  SaturateOnIntegerOverflow=off  RndMeth=Floor
  target_id : Outport
  wires:
  target_frame/1 -> Cast/1
  Cast/1 -> target_id/1

== system NDT_Localization/initial_pose_callback/lookupTransform/if_false/lookupFrameNumber1 ==
  source_frame : Inport
  Cast : DataTypeConversion  OutDataTypeStr=uint32  SaturateOnIntegerOverflow=off  RndMeth=Floor
  source_id : Outport
  wires:
  Cast/1 -> source_id/1
  source_frame/1 -> Cast/1

== system NDT_Localization/initial_pose_callback/lookupTransform/if_false/walkToTopParent ==
  accum : Inport
  time : Inport  Port=2
  target_id : Inport  Port=3
  source_id : Inport  Port=4
  Out1 : Outport

== system NDT_Localization/initial_pose_callback/lookupTransform/if_true/If Action Subsystem ==
  In1 : Inport
  Action Port : ActionPort  ActionPortLabel=else
  Out1 : Outport
  wires:
  In1/1 -> Out1/1

== system NDT_Localization/initial_pose_callback/lookupTransform/if_true/If Action Subsystem1 ==
  cache : Inport
  Action Port : ActionPort  ActionPortLabel=if(u1 == u2)
  Constant : Constant  Commented=on  Value=null
  Constant1 : Constant  Value=true  OutDataTypeStr=boolean
  Constant2 : Constant  Value=false  OutDataTypeStr=boolean
  If : If  NumInputs=2  IfExpression=u1 ~= u2
  If Action Subsystem : Subsystem  TreatAsAtomicUnit=on
  If Action Subsystem1 : Subsystem  TreatAsAtomicUnit=on
  Merge : Merge
  out1 : Outport
  wires:
  Constant/1 -> If/2
  If/1 -> If Action Subsystem/Action
  If/2 -> If Action Subsystem1/Action
  Constant1/1 -> If Action Subsystem/1(In1)
  Constant2/1 -> If Action Subsystem1/1(In1)
  If Action Subsystem/1(Out1) -> Merge/1
  If Action Subsystem1/1(Out1) -> Merge/2
  Merge/1 -> out1/1
  cache/1 -> If/1

== system NDT_Localization/initial_pose_callback/lookupTransform/if_true/getFrame ==
  target_id : Inport
  cache : Outport
  wires:
  target_id/1 -> cache/1

== system NDT_Localization/initial_pose_callback/lookupTransform/if_true/getLatestTimestamp ==
  cache : Inport
  LatestTimestamp : Outport
  wires:
  cache/1 -> LatestTimestamp/1

== system NDT_Localization/initial_pose_callback/lookupTransform/if_true/lookupFrameNumber ==
  target_frame : Inport
  Cast : DataTypeConversion  OutDataTypeStr=uint32  SaturateOnIntegerOverflow=off  RndMeth=Floor
  target_id : Outport
  wires:
  target_frame/1 -> Cast/1
  Cast/1 -> target_id/1

== system NDT_Localization/map_callback/check_localizer/set_map/set_map_impl ==
  msg : Inport
  insert : Subsystem
  m_stamp : Outport
  m_frame_id : Outport  Port=2
  impl() : Outport  Port=3
  Out1 : Outport  Port=4
  wires:
  msg/1 -> insert/1(msg)
  insert/1(m_stamp) -> m_stamp/1
  insert/2(m_frame_id) -> m_frame_id/1
  insert/3(impl()) -> impl()/1
  insert/4(Out1) -> Out1/1

== system NDT_Localization/observation_callback/check_localizer/If Action Subsystem/If Action Subsystem ==
  pose_out : Inport
  ob_msg : Inport  Port=2
  summary : Inport  Port=3
  Action Port : ActionPort  ActionPortLabel=if(u1 ~= 0)
  Constant : Constant
  handle_registration_summary : Subsystem
  msg : Outport
  Out1 : Outport  Port=2
  Out2 : Outport  Port=3
  wires:
  Constant/1 -> Out2/1
  summary/1 -> handle_registration_summary/1(summary)
  pose_out/1 -> Out1/1
  ob_msg/1 -> msg/1

== system NDT_Localization/observation_callback/check_localizer/If Action Subsystem/If Action Subsystem1 ==
  Action Port : ActionPort  ActionPortLabel=else
  Constant : Constant  Value=0
  Out1 : Outport
  wires:
  Constant/1 -> Out1/1

== system NDT_Localization/observation_callback/check_localizer/If Action Subsystem/If Action Subsystem2 ==
  In1 : Inport
  external_pose_available : Inport  Port=2
  initial_guess : Inport  Port=3
  Action Port : ActionPort  ActionPortLabel=if(u1 ~= 0)
  Constant : Constant
  Switch : Switch  Criteria=u2 ~= 0  SaturateOnIntegerOverflow=off  InputSameDT=off
  Out1 : Outport
  Out2 : Outport  Port=2
  wires:
  In1/1 -> Switch/1
  external_pose_available/1 -> Switch/2
  initial_guess/1 -> Switch/3
  Switch/1 -> Out1/1
  Constant/1 -> Out2/1

== system NDT_Localization/observation_callback/check_localizer/If Action Subsystem/guess ==
  observation_time : Inport
  map_frame : Inport  Port=2
  observation_frame : Inport  Port=3
  Switch : Switch  Criteria=u2 ~= 0  SaturateOnIntegerOverflow=off  InputSameDT=off
  extrapolate : Subsystem
  lookupTransform : Subsystem
  initial_guess : Outport
  wires:
  lookupTransform/1(ret) -> Switch/1
  extrapolate/1(Out1) -> Switch/3
  lookupTransform/2(Out1) -> Switch/2
  Switch/1 -> initial_guess/1
  map_frame/1 -> lookupTransform/1(map_frame), extrapolate/2(map_frame)
  observation_frame/1 -> extrapolate/3(observation_frame), lookupTransform/2(observation_frame)
  observation_time/1 -> lookupTransform/3(observation_time), extrapolate/1(observation_time)

== system NDT_Localization/observation_callback/check_localizer/If Action Subsystem/register_measurement_impl ==
  observation_time : Inport
  ob_msg : Inport  Port=2
  ob_msg_data : Inport  Port=3
  initial_guess : Inport  Port=4
  m_map : Inport  Port=5
  m_map.frame_id() : Inport  Port=6
  localizer_ptr : Inport  Port=7
  If Action Subsystem : Subsystem  TreatAsAtomicUnit=on
  If Action Subsystem1 : Subsystem  TreatAsAtomicUnit=on
  Merge : Merge
  validate_msg : Subsystem
  summary : Outport
  pose_out : Outport  Port=2
  Out1 : Outport  Port=3
  wires:
  If Action Subsystem1/1(Out1) -> Merge/2
  If Action Subsystem/3(Out1) -> Merge/1
  Merge/1 -> Out1/1
  ob_msg/1 -> If Action Subsystem/2(ob_msg)
  initial_guess/1 -> If Action Subsystem/4(initial_guess)
  observation_time/1 -> If Action Subsystem/1(message_time), validate_msg/1(observation_time)  "message_time"
  m_map/1 -> If Action Subsystem/6(m_map), validate_msg/2(m_map)
  validate_msg/1(Out1) -> If Action Subsystem/Action
  validate_msg/2(Out2) -> If Action Subsystem1/Action
  m_map.frame_id()/1 -> If Action Subsystem/5(m_map.frame_id())
  ob_msg_data/1 -> If Action Subsystem/3(ob_msg_data)
  If Action Subsystem/1(summary) -> summary/1
  If Action Subsystem/2(pose_out) -> pose_out/1
  localizer_ptr/1 -> If Action Subsystem/7(localizer_ptr)

== system NDT_Localization/observation_callback/check_localizer/If Action Subsystem/validate_output ==
  summary : Inport
  pose_out : Inport  Port=2
  initial_guess : Inport  Port=3
  Data Type Conversion : DataTypeConversion  OutDataTypeStr=uint8  SaturateOnIntegerOverflow=off  RndMeth=Floor
  Data Type Conversion1 : DataTypeConversion  OutDataTypeStr=uint8  SaturateOnIntegerOverflow=off  RndMeth=Floor
  If : If  IfExpression=u1 ~= 0
  If Action Subsystem : Subsystem  TreatAsAtomicUnit=on
  If Action Subsystem1 : Subsystem  TreatAsAtomicUnit=on
  If1 : If  IfExpression=u1 ~= 0
  Merge : Merge  Inputs=3
  Merge1 : Merge
  Merge3 : Merge
  Switch Case : SwitchCase  CaseConditions={2,1}
  Switch Case Action Subsystem : Subsystem  TreatAsAtomicUnit=on
  Switch Case Action Subsystem1 : Subsystem  TreatAsAtomicUnit=on
  Switch Case Action Subsystem2 : Subsystem  TreatAsAtomicUnit=on
  ret_out : Outport
  wires:
  Switch Case/3 -> Switch Case Action Subsystem2/Action
  summary/1 -> Switch Case Action Subsystem1/1(summary)
  Switch Case Action Subsystem/1(ret) -> Merge/1
  Switch Case Action Subsystem1/1(ret) -> Merge/2
  Switch Case Action Subsystem2/1(ret) -> Merge/3
  If/1 -> If Action Subsystem/Action
  If/2 -> Merge1/1
  If Action Subsystem/1(Out1) -> Merge1/2
  Data Type Conversion/1 -> If/1
  Merge/1 -> Data Type Conversion/1
  initial_guess/1 -> Switch Case Action Subsystem1/3(initial_guess), If Action Subsystem1/2(initial_guess), If Action Subsystem/2(initial_guess)
  If Action Subsystem1/1(Out1) -> Merge3/2
  pose_out/1 -> Switch Case Action Subsystem1/2(pose_out), If Action Subsystem1/1(pose_out), If Action Subsystem/1(pose_out)
  Merge1/1 -> Data Type Conversion1/1
  Data Type Conversion1/1 -> If1/1
  If1/2 -> Merge3/1
  If1/1 -> If Action Subsystem1/Action
  Merge3/1 -> ret_out/1
  Switch Case/1 -> Switch Case Action Subsystem/Action
  Switch Case/2 -> Switch Case Action Subsystem1/Action

== system NDT_Localization/observation_callback/check_localizer/If Action Subsystem2/republish_tf ==
  msg.header.stamp : Inport
  m_localizer_ptr : Inport  Port=2
  Bus Selector : BusSelector  OutputSignals=signal1
  Out1 : Outport
  wires:
  msg.header.stamp/1 -> ?
  m_localizer_ptr/1 -> Bus Selector/1
  Bus Selector/1 -> ?  "<signal1>"

== system NDT_Localization/initial_pose_callback/canTransform/else/canTransformNoLock/true ==
  In1 : Inport
  Action Port : ActionPort  ActionPortLabel=if(u1 == u2)
  Out1 : Outport
  wires:
  In1/1 -> Out1/1

== system NDT_Localization/initial_pose_callback/canTransform/else/canTransformNoLock/walkToTopParent ==
  accum : Inport
  time : Inport  Port=2
  target_id : Inport  Port=3
  source_id : Inport  Port=4
  error_msg : Inport  Port=5
  Action Port : ActionPort  ActionPortLabel=else
  Out2 : Outport
  wires:
  ? -> Out2/1

== system NDT_Localization/initial_pose_callback/lookupTransform/if_true/If Action Subsystem1/If Action Subsystem ==
  In1 : Inport
  Action Port : ActionPort  ActionPortLabel=if(u1 ~= u2)
  Out1 : Outport
  wires:
  In1/1 -> Out1/1

== system NDT_Localization/initial_pose_callback/lookupTransform/if_true/If Action Subsystem1/If Action Subsystem1 ==
  In1 : Inport
  Action Port : ActionPort  ActionPortLabel=else
  Out1 : Outport
  wires:
  In1/1 -> Out1/1

== system NDT_Localization/map_callback/check_localizer/set_map/set_map_impl/insert ==
  msg : Inport
  Add : Sum
  Bus Selector : BusSelector  OutputSignals=header.stamp.sec,header.stamp.nanosec,header.frame_id
  Constant1 : Constant  Value=0.001
  Constant2 : Constant  Value=9
  Math Function : Math  Operator=10^u
  Product : Product  OutDataTypeStr=uint32
  Product1 : Product
  insert_ : Subsystem
  m_stamp : Outport
  m_frame_id : Outport  Port=2
  impl() : Outport  Port=3
  Out1 : Outport  Port=4
  wires:
  msg/1 -> insert_/1(msg), Bus Selector/1
  Add/1 -> Product1/1
  Bus Selector/1 -> Product/2  "<sec>"
  Math Function/1 -> Product/1
  Bus Selector/2 -> Add/2  "<nanosec>"
  Product/1 -> Add/1
  Bus Selector/3 -> m_frame_id/1  "<frame_id>"
  Product1/1 -> m_stamp/1  "stamp"
  Constant1/1 -> Product1/2
  insert_/1(insert_res) -> impl()/1
  insert_/2(Out2) -> Out1/1
  Constant2/1 -> Math Function/1

== system NDT_Localization/observation_callback/check_localizer/If Action Subsystem/If Action Subsystem/handle_registration_summary ==
  summary : Inport
  Data Type Conversion : DataTypeConversion  OutDataTypeStr=uint8  SaturateOnIntegerOverflow=off  RndMeth=Floor
  If : If  IfExpression=u1 ~= 0  ShowElse=off
  If Action Subsystem : Subsystem  TreatAsAtomicUnit=on
  wires:
  summary/1 -> Data Type Conversion/1, If Action Subsystem/1(summary)
  If/1 -> If Action Subsystem/Action
  Data Type Conversion/1 -> If/1

== system NDT_Localization/observation_callback/check_localizer/If Action Subsystem/guess/extrapolate ==
  observation_time : Inport
  map_frame : Inport  Port=2
  observation_frame : Inport  Port=3
  Add : Sum
  Bus Selector : BusSelector  OutputSignals=header.stamp.sec,header.stamp.nanosec
  Constant : Constant  Value=9
  Data Type Conversion : DataTypeConversion  OutDataTypeStr=uint8  SaturateOnIntegerOverflow=off  RndMeth=Floor
  If : If  IfExpression=u1 ~= 0  ShowElse=off
  If Action Subsystem1 : Subsystem  TreatAsAtomicUnit=on
  Math Function : Math  Operator=10^u
  Product : Product
  Relational Operator : RelationalOperator  Operator=<=  OutDataTypeStr=boolean  RndMeth=Simplest  InputSameDT=off
  lookupTransform : Subsystem
  Out1 : Outport
  wires:
  If/1 -> If Action Subsystem1/Action
  If Action Subsystem1/1(Out2) -> Out1/1
  Product/1 -> Add/1
  Bus Selector/2 -> Add/2  "<nanosec>"
  Constant/1 -> Math Function/1
  Bus Selector/1 -> Product/1  "<sec>"
  lookupTransform/1(ret) -> If Action Subsystem1/1(ret), Bus Selector/1
  Math Function/1 -> Product/2
  Add/1 -> Relational Operator/1  "observation_time"
  Relational Operator/1 -> Data Type Conversion/1
  Data Type Conversion/1 -> If/1
  observation_time/1 -> Relational Operator/2
  map_frame/1 -> lookupTransform/1(map_frame)
  observation_frame/1 -> lookupTransform/2(observation_frame)

== system NDT_Localization/observation_callback/check_localizer/If Action Subsystem/guess/lookupTransform ==
  map_frame : Inport
  observation_frame : Inport  Port=2
  observation_time : Inport  Port=3
  Constant : Constant
  If : If  IfExpression=u1 ~= 0
  String Compare : StringCompare
  Switch : Switch  Criteria=u2 > Threshold  SaturateOnIntegerOverflow=off  InputSameDT=off
  if_false : Subsystem  TreatAsAtomicUnit=on
  if_true : Subsystem  TreatAsAtomicUnit=on
  ret : Outport
  Out1 : Outport  Port=2
  wires:
  Constant/1 -> Out1/1
  Switch/1 -> ret/1
  map_frame/1 -> String Compare/1, if_false/1(target_frame), if_true/1(target_frame)
  if_true/1(identity) -> Switch/1
  observation_time/1 -> if_false/3(time), if_true/3(time)
  If/1 -> if_true/Action
  String Compare/1 -> Switch/2, If/1
  if_false/1(output_transform) -> Switch/3
  If/2 -> if_false/Action
  observation_frame/1 -> String Compare/2, if_false/2(source_frame), if_true/2(source_frame)
